simulink model "PreBraking_Scenario1_cs"  (R2014b)
settings: Solver=ode5  SolverMode=SingleTasking  StartTime=0.0  StopTime=inf  FixedStep=1/100  RelTol=1e-3
PreLoadFcn:
  | mbxruntime.callbacks.PreLoadFcn(bdroot);
  | check_NUTS_defined;
  | 
  | assignin('base',['model_closed_' bdroot],false);addpath('../includes_AEBS');
PostLoadFcn:
  | mbxruntime.callbacks.PostLoadFcn(bdroot);
InitFcn:
  | mbxruntime.callbacks.InitFcn(bdroot);
StartFcn:
  | mbxruntime.callbacks.StartFcn(bdroot);
StopFcn:
  | mbxruntime.callbacks.StopFcn(bdroot);
model workspace: external: MAT-File .\PreBraking_Scenario1_cs_hws.mat (data not in the file)
undefined symbols (not defined in the file or in its folder): OrientationPitch, OrientationRoll, PositionX, PositionY, PositionZ, warningInitialVelocity, x0
undefined symbols (not defined in the file): PreBraking_Scenario1_cs_026d0cdcec288b62, PreBraking_Scenario1_cs_0385b51e7df15a58, PreBraking_Scenario1_cs_0b30baef7b6532db, PreBraking_Scenario1_cs_0d6875a57991286b, PreBraking_Scenario1_cs_138be516424db58b, PreBraking_Scenario1_cs_23d3d4fc5b63e353, PreBraking_Scenario1_cs_2f0f014f8afaa95e, PreBraking_Scenario1_cs_37a5b238ce9b9d58, PreBraking_Scenario1_cs_3e434e556dc94cce, PreBraking_Scenario1_cs_46f0ee8501fe1889, PreBraking_Scenario1_cs_5d62597554acff95, PreBraking_Scenario1_cs_5da0fc6e87d9d5b3, PreBraking_Scenario1_cs_5ed65167116c3469, PreBraking_Scenario1_cs_6eb9f15635d94d0c, PreBraking_Scenario1_cs_783b9a4fac440b07, PreBraking_Scenario1_cs_7a7290d742a44883, PreBraking_Scenario1_cs_82e3a60ee2034171, PreBraking_Scenario1_cs_8b2784fe49c992e6, PreBraking_Scenario1_cs_9206a2e3911d44de, PreBraking_Scenario1_cs_983f811fe80a5f0d, PreBraking_Scenario1_cs_9b466beab5d2337e, PreBraking_Scenario1_cs_a08e42c00c044b50, PreBraking_Scenario1_cs_Audi_A8_1_Dynamics_Simple_initialPitch, PreBraking_Scenario1_cs_Audi_A8_1_Dynamics_Simple_initialRoll, PreBraking_Scenario1_cs_Audi_A8_1_Dynamics_Simple_initialX, PreBraking_Scenario1_cs_Audi_A8_1_Dynamics_Simple_initialY, PreBraking_Scenario1_cs_Audi_A8_1_Dynamics_Simple_initialYaw, PreBraking_Scenario1_cs_Audi_A8_1_Dynamics_Simple_initialZ, PreBraking_Scenario1_cs_b7d11204e3bec466, PreBraking_Scenario1_cs_c7aafe2117783533, PreBraking_Scenario1_cs_cbbde59a5a2cb59b, PreBraking_Scenario1_cs_ccf63f357a330662, PreBraking_Scenario1_cs_Citroen_C3_3_Path_pathUniqueID, PreBraking_Scenario1_cs_d4efba4491f01d46, PreBraking_Scenario1_cs_d59dc65fc07c1f25, PreBraking_Scenario1_cs_d8dfcf69a768aef8, PreBraking_Scenario1_cs_dcfa2001fd35d12a, PreBraking_Scenario1_cs_eaed30225f637059, PreBraking_Scenario1_cs_ecfe80b42161c93b, PreBraking_Scenario1_cs_f61ea707e711400d, PreBraking_Scenario1_cs_Toyota_Previa_1_Path_pathUniqueID, SteeringColumn, SteeringWheel, WheelL0, WheelL1, WheelR0, WheelR1
libraries: simulink_extras x41, simulink x20, PreScanSimulinkLibrary x13, PreScanUsefulBlocks x2
(part 1 of 14)
CloseFcn:
  | mbxruntime.callbacks.CloseFcn(bdroot);
  | evalin('base',['clear model_closed_' bdroot]);
settings Model: Creator=PRESCAN  LastModifiedBy=jenkins
settings DataIOCC: SignalLoggingSaveFormat=ModelDataLogs
settings OptimizationCC: InlineParams=on  ExpressionDepthLimit=2147483647  InitFltsAndDblsToZero=on
settings DebuggingCC: SaveWithParameterizedLinksMsg=none  UnderspecifiedInitializationDetection=Classic  MergeDetectMultiDrivingBlocksExec=none  SignalResolutionControl=TryResolveAllWithWarning  SolverPrmCheckMsg=none  MultiTaskDSMMsg=warning  MultiTaskCondExecSysMsg=none  FcnCallInpInsideContextMsg=UseLocalSettings  StateNameClashWarn=warning
settings ModelReferenceCC: UpdateModelReferenceTargets=IfOutOfDate
settings SFSimCC: SimParseCustomCode=off
settings SFSimCC: SimCustomHeaderCode=|
  | #include "prescan_collisiondetection_data.h"
  | #include "prescan.h"
  | #include "prescan_platform.h"
settings RTWCC: IncludeERTFirstTime=on
settings GRTTargetCC: TargetFcnLib=ansi_tfl_tmw.mat  CombineOutputUpdateFcns=off  GRTInterface=on

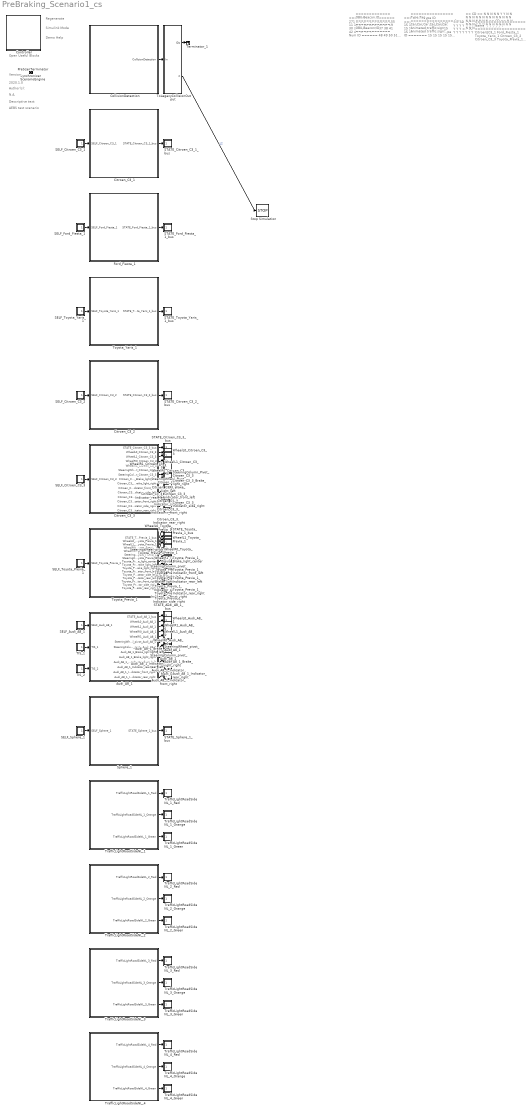
== system PreBraking_Scenario1_cs ==
  note: Regenerate
  note: Simulink Mode
  note: Open Useful Blocks
  note: 2020.1.0
  note: Version:
  note: Author(s):
  note: N.A.
  note: Descriptive text:
  note: AEBS test scenario
  note: Demo Help
  note: ======
      | Num ID
      | ======
      | 271
      | 272
      | 274
      | 276
      | 152
      | 18
      | 155
      | 11
      | 13
      | 14
      | 15
      | 21
      | 24
      | 26
      | 27
      | 29
      | 30
      | 31
      | 32
      | 33
      | 34
      | 35
      | 37
      | 38
      | 41
      | 42
      | 44
      | 45
      | 46
      | 47
      | ======
      | Num ID
      | ======
      | 48
      | 49
      | 50
      | 51
      | 52
      | 54
      | 55
      | 180
      | 188
      | 196
      | 204
      | 210
      | 218
      | 226
      | 234
      | 579
      | 586
      | 591
      | 154
  note: =============
      | OBU-Beacon ID
      | =============
      |
      |
      |
      |
      |
      |
      |
      |
      |
      |
      |
      |
      |
      |
      |
      |
      |
      |
      |
      |
      |
      |
      |
      |
      |
      |
      |
      |
      |
      |
      | =============
      | OBU-Beacon ID
      | =============
  note: =======
      | Type ID
      | =======
      | 1
      | 1
      | 1
      | 1
      | 1
      | 1
      | 1
      | 15
      | 15
      | 15
      | 15
      | 15
      | 15
      | 15
      | 15
      | 15
      | 15
      | 15
      | 15
      | 15
      | 15
      | 15
      | 15
      | 15
      | 15
      | 15
      | 15
      | 15
      | 15
      | 15
      | =======
      | Type ID
      | =======
      | 15
      | 15
      | 15
      | 15
      | 15
      | 15
      | 15
      | 13
      | 13
      | 13
      | 13
      | 13
      | 13
      | 13
      | 13
      | 13
      | 13
      | 13
      | 13
  note: ================
      | Type Tag
      | ================
      | Car
      | Car
      | Car
      | Car
      | Car
      | Car
      | Car
      | Animated traffic sign
      | Animated traffic sign
      | Animated traffic sign
      | Animated traffic sign
      | Animated traffic sign
      | Animated traffic sign
      | Animated traffic sign
      | Animated traffic sign
      | Animated traffic sign
      | Animated traffic sign
      | Animated traffic sign
      | Animated traffic sign
      | Animated traffic sign
      | Animated traffic sign
      | Animated traffic sign
      | Animated traffic sign
      | Animated traffic sign
      | Animated traffic sign
      | Animated traffic sign
      | Animated traffic sign
      | Animated traffic sign
      | Animated traffic sign
      | Animated traffic sign
      | ================
      | Type Tag
      | ================
      | Animated traffic sign
      | Animated traffic sign
      | Animated traffic sign
      | Animated traffic sign
      | Animated traffic sign
      | Animated traffic sign
      | Animated traffic sign
      | Natural element
      | Natural element
      | Natural element
      | Natural element
      | Natural element
      | Natural element
      | Natural element
      | Natural element
      | Natural element
      | Natural element
      | Natural element
      | Natural element
  note: ==
      | SD
      | ==
      | Y
      | Y
      | Y
      | Y
      | Y
      | Y
      | Y
      | Y
      | Y
      | Y
      | Y
      | Y
      | Y
      | Y
      | Y
      | Y
      | Y
      | Y
      | Y
      | Y
      | Y
      | Y
      | Y
      | Y
      | Y
      | Y
      | Y
      | Y
      | Y
      | Y
      | ==
      | SD
      | ==
      | Y
      | Y
      | Y
      | Y
      | Y
      | Y
      | Y
      | Y
      | Y
      | Y
      | Y
      | Y
      | Y
      | Y
      | Y
      | Y
      | Y
      | Y
      | Y
  note: ==
      | CD
      | ==
      | N
      | N
      | N
      | N
      | N
      | Y
      | Y
      | N
      | N
      | N
      | N
      | N
      | N
      | N
      | N
      | N
      | N
      | N
      | N
      | N
      | N
      | N
      | N
      | N
      | N
      | N
      | N
      | N
      | N
      | N
      | ==
      | CD
      | ==
      | N
      | N
      | N
      | N
      | N
      | N
      | N
      | N
      | N
      | N
      | N
      | N
      | N
      | N
      | N
      | N
      | N
      | N
      | N
  note: ===================
      | Name
      | ===================
      | Citroen_C3_1
      | Ford_Fiesta_1
      | Toyota_Yaris_1
      | Citroen_C3_2
      | Citroen_C3_3
      | Toyota_Previa_1
      | Audi_A8_1
      | TrafficLightRoadSideNL_1
      | TrafficLightRoadSideNL_2
      | TrafficLightRoadSideNL_3
      | TrafficLightRoadSideNL_4
      | Lightpost_1
      | Lightpost_3
      | Lightpost_5
      | Lightpost_6
      | Lightpost_8
      | Lightpost_9
      | Lightpost_10
      | Lightpost_11
      | Lightpost_12
      | Lightpost_13
      | Lightpost_14
      | Lightpost_16
      | Lightpost_17
      | Lightpost_20
      | Lightpost_21
      | Lightpost_23
      | Lightpost_24
      | Lightpost_25
      | Lightpost_26
      | ===================
      | Name
      | ===================
      | Lightpost_27
      | Lightpost_28
      | Lightpost_29
      | Lightpost_30
      | Lightpost_31
      | Lightpost_33
      | Lightpost_34
      | ServiceBerry_Age12_31
      | ServiceBerry_Age12_39
      | ServiceBerry_Age12_47
      | ServiceBerry_Age12_55
      | ServiceBerry_Age12_61
      | ServiceBerry_Age12_69
      | ServiceBerry_Age12_77
      | ServiceBerry_Age12_85
      | ServiceBerry_Age12_430
      | ServiceBerry_Age12_437
      | ServiceBerry_Age12_442
      | Magnolia_Age10_1
  Audi_A8_1 : Subsystem  Tag=WorldObjectSubSystem  InitFcn=UniqueId = '1001';
      mask init:
      | modelPath = GenericModelHelper.getGenericModelFilePath('ModelDepo','Vehicles\Audi_A8\Audi_A8.pgmb','e33fe1ddcf3e8ae97caccbc8f2fa74ac');imagePath = GenericModelHelper.getCompilationPicture(modelPath, 'Audi_A8_HighPoly.png');
      mask Display: image(imread(imagePath));color('white');text(0, 0, ' ID=155\n')
  Audi_A8_1_Brake_light_left : Subsystem  Tag=actuator/BrakeLightL  Priority=0  LoadFcn=load('PreScanVisuLightActuatorData');load('PrescanRPYData');load('PrescanXYZData');load('PreScanRGBData')  mask(PreScan Sink Block: VisuActiveLight){}
      mask help:
      | The VisuActiveLight block provides a way for detailed animation of Light Sources, such as the indicator, brake, fog and main lights of a vehicle, or a light post.
      |
      | For more information, please click Help.
      settings: OpenFcn=open_system([gcb '/Actuator'],'mask')
      mask Help: eval('openHelp(209)')
      mask Display: image(imread('HeadLight.png'))
  Audi_A8_1_Brake_light_right : Subsystem  Tag=actuator/BrakeLightR  Priority=0  LoadFcn=load('PreScanVisuLightActuatorData');load('PrescanRPYData');load('PrescanXYZData');load('PreScanRGBData')  mask(PreScan Sink Block: VisuActiveLight){}
      mask help:
      | The VisuActiveLight block provides a way for detailed animation of Light Sources, such as the indicator, brake, fog and main lights of a vehicle, or a light post.
      |
      | For more information, please click Help.
      settings: OpenFcn=open_system([gcb '/Actuator'],'mask')
      mask Help: eval('openHelp(209)')
      mask Display: image(imread('HeadLight.png'))
  Audi_A8_1_Indicator_front_left : Subsystem  Tag=actuator/IndicatorFL  Priority=0  LoadFcn=load('PreScanVisuLightActuatorData');load('PrescanRPYData');load('PrescanXYZData');load('PreScanRGBData')  mask(PreScan Sink Block: VisuActiveLight){}
      mask help:
      | The VisuActiveLight block provides a way for detailed animation of Light Sources, such as the indicator, brake, fog and main lights of a vehicle, or a light post.
      |
      | For more information, please click Help.
      settings: OpenFcn=open_system([gcb '/Actuator'],'mask')
      mask Help: eval('openHelp(209)')
      mask Display: image(imread('HeadLight.png'))
  Audi_A8_1_Indicator_front_right : Subsystem  Tag=actuator/IndicatorFR  Priority=0  LoadFcn=load('PreScanVisuLightActuatorData');load('PrescanRPYData');load('PrescanXYZData');load('PreScanRGBData')  mask(PreScan Sink Block: VisuActiveLight){}
      mask help:
      | The VisuActiveLight block provides a way for detailed animation of Light Sources, such as the indicator, brake, fog and main lights of a vehicle, or a light post.
      |
      | For more information, please click Help.
      settings: OpenFcn=open_system([gcb '/Actuator'],'mask')
      mask Help: eval('openHelp(209)')
      mask Display: image(imread('HeadLight.png'))
  Audi_A8_1_Indicator_rear_left : Subsystem  Tag=actuator/IndicatorRL  Priority=0  LoadFcn=load('PreScanVisuLightActuatorData');load('PrescanRPYData');load('PrescanXYZData');load('PreScanRGBData')  mask(PreScan Sink Block: VisuActiveLight){}
      mask help:
      | The VisuActiveLight block provides a way for detailed animation of Light Sources, such as the indicator, brake, fog and main lights of a vehicle, or a light post.
      |
      | For more information, please click Help.
      settings: OpenFcn=open_system([gcb '/Actuator'],'mask')
      mask Help: eval('openHelp(209)')
      mask Display: image(imread('HeadLight.png'))
  Audi_A8_1_Indicator_rear_right : Subsystem  Tag=actuator/IndicatorRR  Priority=0  LoadFcn=load('PreScanVisuLightActuatorData');load('PrescanRPYData');load('PrescanXYZData');load('PreScanRGBData')  mask(PreScan Sink Block: VisuActiveLight){}
      mask help:
      | The VisuActiveLight block provides a way for detailed animation of Light Sources, such as the indicator, brake, fog and main lights of a vehicle, or a light post.
      |
      | For more information, please click Help.
      settings: OpenFcn=open_system([gcb '/Actuator'],'mask')
      mask Help: eval('openHelp(209)')
      mask Display: image(imread('HeadLight.png'))
  Citroen_C3_1 : Subsystem  Tag=WorldObjectSubSystem  InitFcn=UniqueId = '978';
      mask init:
      | modelPath = GenericModelHelper.getGenericModelFilePath('ModelDepo','Vehicles\Citroen_C3\Citroen_C3.pgmb','e804ced06d50dbfc6a2202ab3ad01b0c');imagePath = GenericModelHelper.getCompilationPicture(modelPath, 'Citroen_C3_HighPoly.png');
      mask Display: image(imread(imagePath));color('white');text(0, 0, ' ID=271\n')
  Citroen_C3_2 : Subsystem  Tag=WorldObjectSubSystem  InitFcn=UniqueId = '981';
      mask init: same as PreBraking_Scenario1_cs/Citroen_C3_1
      mask Display: image(imread(imagePath));color('white');text(0, 0, ' ID=276\n')
  Citroen_C3_3 : Subsystem  Tag=WorldObjectSubSystem  InitFcn=UniqueId = '987';
      mask init: same as PreBraking_Scenario1_cs/Citroen_C3_1
      mask Display: image(imread(imagePath));color('white');text(0, 0, ' ID=152\n')
  Citroen_C3_3_Brake_light_left : Subsystem  Tag=actuator/BrakeLightL_Pivot  Priority=0  LoadFcn=load('PreScanVisuLightActuatorData');load('PrescanRPYData');load('PrescanXYZData');load('PreScanRGBData')  mask(PreScan Sink Block: VisuActiveLight){}
      mask help:
      | The VisuActiveLight block provides a way for detailed animation of Light Sources, such as the indicator, brake, fog and main lights of a vehicle, or a light post.
      |
      | For more information, please click Help.
      settings: OpenFcn=open_system([gcb '/Actuator'],'mask')
      mask Help: eval('openHelp(209)')
      mask Display: image(imread('HeadLight.png'))
  Citroen_C3_3_Brake_light_right : Subsystem  Tag=actuator/BrakeLightR_Pivot  Priority=0  LoadFcn=load('PreScanVisuLightActuatorData');load('PrescanRPYData');load('PrescanXYZData');load('PreScanRGBData')  mask(PreScan Sink Block: VisuActiveLight){}
      mask help:
      | The VisuActiveLight block provides a way for detailed animation of Light Sources, such as the indicator, brake, fog and main lights of a vehicle, or a light post.
      |
      | For more information, please click Help.
      settings: OpenFcn=open_system([gcb '/Actuator'],'mask')
      mask Help: eval('openHelp(209)')
      mask Display: image(imread('HeadLight.png'))
  Citroen_C3_3_Indicator_front_left : Subsystem  Tag=actuator/IndicatorFL_Pivot  Priority=0  LoadFcn=load('PreScanVisuLightActuatorData');load('PrescanRPYData');load('PrescanXYZData');load('PreScanRGBData')  mask(PreScan Sink Block: VisuActiveLight){}
      mask help:
      | The VisuActiveLight block provides a way for detailed animation of Light Sources, such as the indicator, brake, fog and main lights of a vehicle, or a light post.
      |
      | For more information, please click Help.
      settings: OpenFcn=open_system([gcb '/Actuator'],'mask')
      mask Help: eval('openHelp(209)')
      mask Display: image(imread('HeadLight.png'))
  Citroen_C3_3_Indicator_front_right : Subsystem  Tag=actuator/IndicatorFR_Pivot  Priority=0  LoadFcn=load('PreScanVisuLightActuatorData');load('PrescanRPYData');load('PrescanXYZData');load('PreScanRGBData')  mask(PreScan Sink Block: VisuActiveLight){}
      mask help:
      | The VisuActiveLight block provides a way for detailed animation of Light Sources, such as the indicator, brake, fog and main lights of a vehicle, or a light post.
      |
      | For more information, please click Help.
      settings: OpenFcn=open_system([gcb '/Actuator'],'mask')
      mask Help: eval('openHelp(209)')
      mask Display: image(imread('HeadLight.png'))
  Citroen_C3_3_Indicator_rear_left : Subsystem  Tag=actuator/IndicatorRL_Pivot  Priority=0  LoadFcn=load('PreScanVisuLightActuatorData');load('PrescanRPYData');load('PrescanXYZData');load('PreScanRGBData')  mask(PreScan Sink Block: VisuActiveLight){}
      mask help:
      | The VisuActiveLight block provides a way for detailed animation of Light Sources, such as the indicator, brake, fog and main lights of a vehicle, or a light post.
      |
      | For more information, please click Help.
      settings: OpenFcn=open_system([gcb '/Actuator'],'mask')
      mask Help: eval('openHelp(209)')
      mask Display: image(imread('HeadLight.png'))
  Citroen_C3_3_Indicator_rear_right : Subsystem  Tag=actuator/IndicatorRR_Pivot  Priority=0  LoadFcn=load('PreScanVisuLightActuatorData');load('PrescanRPYData');load('PrescanXYZData');load('PreScanRGBData')  mask(PreScan Sink Block: VisuActiveLight){}
      mask help:
      | The VisuActiveLight block provides a way for detailed animation of Light Sources, such as the indicator, brake, fog and main lights of a vehicle, or a light post.
      |
      | For more information, please click Help.
      settings: OpenFcn=open_system([gcb '/Actuator'],'mask')
      mask Help: eval('openHelp(209)')
      mask Display: image(imread('HeadLight.png'))
  Citroen_C3_3_Indicator_side_left : Subsystem  Tag=actuator/IndicatorSL_Pivot  Priority=0  LoadFcn=load('PreScanVisuLightActuatorData');load('PrescanRPYData');load('PrescanXYZData');load('PreScanRGBData')  mask(PreScan Sink Block: VisuActiveLight){}
      mask help:
      | The VisuActiveLight block provides a way for detailed animation of Light Sources, such as the indicator, brake, fog and main lights of a vehicle, or a light post.
      |
      | For more information, please click Help.
      settings: OpenFcn=open_system([gcb '/Actuator'],'mask')
      mask Help: eval('openHelp(209)')
      mask Display: image(imread('HeadLight.png'))
  Citroen_C3_3_Indicator_side_right : Subsystem  Tag=actuator/IndicatorSR_Pivot  Priority=0  LoadFcn=load('PreScanVisuLightActuatorData');load('PrescanRPYData');load('PrescanXYZData');load('PreScanRGBData')  mask(PreScan Sink Block: VisuActiveLight){}
      mask help:
      | The VisuActiveLight block provides a way for detailed animation of Light Sources, such as the indicator, brake, fog and main lights of a vehicle, or a light post.
      |
      | For more information, please click Help.
      settings: OpenFcn=open_system([gcb '/Actuator'],'mask')
      mask Help: eval('openHelp(209)')
      mask Display: image(imread('HeadLight.png'))
  CollisionDetection : Subsystem  Tag=sensor/CollisionDetection  Priority=30  LoadFcn=load('PrescanCollisionDetectionData.mat');load('PrescanCollisionDetectionMessage.mat')  mask(PreScan Source Block: CollisionDetection){}
      mask help: Collision Detection can be used to detect collisions between PreScan components. For Collision Detection the actual component shape is taken into account, so it is not a bounding box approach.
      settings: OpenFcn=open_system([gcb '/Sensor'],'mask')
      mask Help: eval('openHelp(811)')
      mask Display: image(imread('crash.jpg'))
  Controller : Subsystem  Description=8A3CD2955739A82C886C20AE3E253D78460D53180EE2C1B14CC08DF75A70BE77  Priority=-1  LoadFcn=load PreScanControllerData  mask(PreScan Simulation Controller){prescanversion='2020.1.0', ModelReferencing=off, TimeStep=1/100, ControlMode=0, PreScanExecutionMode=on, ControllerCount=0, ControllerIndex=0, ControllerOptions=''}
      mask prompts: prescanversion "PreScan Version"; ModelReferencing "Use Model Referencing"; TimeStep "Upload Period [s]"; ControlMode "Control Mode"; PreScanExecutionMode "Execution Mode"; ControllerCount "Controller Count"; ControllerIndex "Controller Index"; ControllerOptions "Controller Options"
      mask help:
      | Please do not remove this block from the compilation sheet,
      | as it connects the model to the PreScan environment.
      mask init:
      | model = bdroot(gcb);
      | ExperimentFile = mbxruntime.findExperimentFile(model,true); %relative path
      | 
      | [d1, d2, d3, prescandata] = prescan_Settings();
      | ModelDepo = fullfile(prescandata,'ModelDepo'); 
      | 
      | RTmode = mbxruntime.getRTMode(model);
      | 
      | SimulationMode = get_param(bdroot,'SimulationMode');
      | if strcmp(SimulationMode, 'rapid-accelerator')
      |     SimulationMode = 'external';
      | end
      | TargetName = get_param(bdroot,'SystemTargetFile');
      settings: ModelCloseFcn=assignin('base',['model_closed_' bdroot],true);
      mask Help: eval('openHelp(812)')
      mask Display: image(imread('prescanlogo.ico'))
  Ford_Fiesta_1 : Subsystem  Tag=WorldObjectSubSystem  InitFcn=UniqueId = '979';
      mask init:
      | modelPath = GenericModelHelper.getGenericModelFilePath('ModelDepo','Vehicles\Ford_Fiesta\Ford_Fiesta.pgmb','fe2c7a73e0a60cba76689b71cd1bb76a');imagePath = GenericModelHelper.getCompilationPicture(modelPath, 'Ford_Fiesta_HighPoly.png');
      mask Display: image(imread(imagePath));color('white');text(0, 0, ' ID=272\n')
  PreScanTerminator : Subsystem  Tag=PreScanTerminator  Priority=999  LoadFcn=load PrescanTerminatorData  mask(PreScan Simulation Terminator){TimeStep=1/100}
      mask prompts: TimeStep "Upload Period [s]"
      mask help:
      | Please do not remove this block from the compilation sheet as it
      | connects the model to the PreScan environment.
      mask Help: eval('openHelp(812)')
      mask Display: image(imread('prescanlogo.ico'))
  SELF_Audi_A8_1 : Subsystem  Tag=sensor/SelfPort  Priority=30  LoadFcn=load('PreScanSelfSensorData.mat')  mask(PreScan Source Block: SELF){}
      mask help:
      | The SELF port shows (state) information of the actor itself. The outputs are position in the experiment's axis system and the GPS coordinates, and the object's absolute velocity and compass heading.
      |
      | For more information, please click Help.
      settings: OpenFcn=open_system([gcb '/Sensor'],'mask')
      mask Help: eval('openHelp(462)')
      mask Display: image(imread('GPS.png'))
  SELF_Citroen_C3_1 : Subsystem  Tag=sensor/SelfPort  Priority=30  LoadFcn=load('PreScanSelfSensorData.mat')  mask(PreScan Source Block: SELF){}
      mask help:
      | The SELF port shows (state) information of the actor itself. The outputs are position in the experiment's axis system and the GPS coordinates, and the object's absolute velocity and compass heading.
      |
      | For more information, please click Help.
      settings: OpenFcn=open_system([gcb '/Sensor'],'mask')
      mask Help: eval('openHelp(462)')
      mask Display: image(imread('GPS.png'))
  SELF_Citroen_C3_2 : Subsystem  Tag=sensor/SelfPort  Priority=30  LoadFcn=load('PreScanSelfSensorData.mat')  mask(PreScan Source Block: SELF){}
      mask help:
      | The SELF port shows (state) information of the actor itself. The outputs are position in the experiment's axis system and the GPS coordinates, and the object's absolute velocity and compass heading.
      |
      | For more information, please click Help.
      settings: OpenFcn=open_system([gcb '/Sensor'],'mask')
      mask Help: eval('openHelp(462)')
      mask Display: image(imread('GPS.png'))
  SELF_Citroen_C3_3 : Subsystem  Tag=sensor/SelfPort  Priority=30  LoadFcn=load('PreScanSelfSensorData.mat')  mask(PreScan Source Block: SELF){}
      mask help:
      | The SELF port shows (state) information of the actor itself. The outputs are position in the experiment's axis system and the GPS coordinates, and the object's absolute velocity and compass heading.
      |
      | For more information, please click Help.
      settings: OpenFcn=open_system([gcb '/Sensor'],'mask')
      mask Help: eval('openHelp(462)')
      mask Display: image(imread('GPS.png'))
  SELF_Ford_Fiesta_1 : Subsystem  Tag=sensor/SelfPort  Priority=30  LoadFcn=load('PreScanSelfSensorData.mat')  mask(PreScan Source Block: SELF){}
      mask help:
      | The SELF port shows (state) information of the actor itself. The outputs are position in the experiment's axis system and the GPS coordinates, and the object's absolute velocity and compass heading.
      |
      | For more information, please click Help.
      settings: OpenFcn=open_system([gcb '/Sensor'],'mask')
      mask Help: eval('openHelp(462)')
      mask Display: image(imread('GPS.png'))
  SELF_Sphere_1 : Subsystem  Tag=sensor/SelfPort  Priority=30  LoadFcn=load('PreScanSelfSensorData.mat')  mask(PreScan Source Block: SELF){}
      mask help:
      | The SELF port shows (state) information of the actor itself. The outputs are position in the experiment's axis system and the GPS coordinates, and the object's absolute velocity and compass heading.
      |
      | For more information, please click Help.
      settings: OpenFcn=open_system([gcb '/Sensor'],'mask')
      mask Help: eval('openHelp(462)')
      mask Display: image(imread('GPS.png'))
  SELF_Toyota_Previa_1 : Subsystem  Tag=sensor/SelfPort  Priority=30  LoadFcn=load('PreScanSelfSensorData.mat')  mask(PreScan Source Block: SELF){}
      mask help:
      | The SELF port shows (state) information of the actor itself. The outputs are position in the experiment's axis system and the GPS coordinates, and the object's absolute velocity and compass heading.
      |
      | For more information, please click Help.
      settings: OpenFcn=open_system([gcb '/Sensor'],'mask')
      mask Help: eval('openHelp(462)')
      mask Display: image(imread('GPS.png'))
  SELF_Toyota_Yaris_1 : Subsystem  Tag=sensor/SelfPort  Priority=30  LoadFcn=load('PreScanSelfSensorData.mat')  mask(PreScan Source Block: SELF){}
      mask help:
      | The SELF port shows (state) information of the actor itself. The outputs are position in the experiment's axis system and the GPS coordinates, and the object's absolute velocity and compass heading.
      |
      | For more information, please click Help.
      settings: OpenFcn=open_system([gcb '/Sensor'],'mask')
      mask Help: eval('openHelp(462)')
      mask Display: image(imread('GPS.png'))
  STATE_Audi_A8_1_bus : Subsystem  Tag=actuator/StatePort  Priority=0  LoadFcn=load('PreScanStateActuatorData.mat')  mask(PreScan Sink Block: State){}
      mask help:
      | The Actor State contains a vector signal of size (9x1), containing the following signals:
      |
      | -  Position    	(x,y,z)             	[m]
      | -  Velocity    	(vx,vy,vz)         	[m/s]
      | -  Angles       	(Roll, Pitch, Yaw)	[rad]
      |
      | The Actor state is defined in the global axis system.
      | The state is superponed on the Initial position defined in the GUI.
      |
      | For more information, please click Help.
      settings: OpenFcn=open_system([gcb '/Actuator'],'mask')
      mask Help: eval('openHelp(222)')
      mask Display: image(imread('State.png'))
  STATE_Citroen_C3_1_bus : Subsystem  Tag=actuator/StatePort  Priority=0  LoadFcn=load('PreScanStateActuatorData.mat')  mask(PreScan Sink Block: State){}
      mask help:
      | The Actor State contains a vector signal of size (9x1), containing the following signals:
      |
      | -  Position    	(x,y,z)             	[m]
      | -  Velocity    	(vx,vy,vz)         	[m/s]
      | -  Angles       	(Roll, Pitch, Yaw)	[rad]
      |
      | The Actor state is defined in the global axis system.
      | The state is superponed on the Initial position defined in the GUI.
      |
      | For more information, please click Help.
      settings: OpenFcn=open_system([gcb '/Actuator'],'mask')
      mask Help: eval('openHelp(222)')
      mask Display: image(imread('State.png'))
  STATE_Citroen_C3_2_bus : Subsystem  Tag=actuator/StatePort  Priority=0  LoadFcn=load('PreScanStateActuatorData.mat')  mask(PreScan Sink Block: State){}
      mask help:
      | The Actor State contains a vector signal of size (9x1), containing the following signals:
      |
      | -  Position    	(x,y,z)             	[m]
      | -  Velocity    	(vx,vy,vz)         	[m/s]
      | -  Angles       	(Roll, Pitch, Yaw)	[rad]
      |
      | The Actor state is defined in the global axis system.
      | The state is superponed on the Initial position defined in the GUI.
      |
      | For more information, please click Help.
      settings: OpenFcn=open_system([gcb '/Actuator'],'mask')
      mask Help: eval('openHelp(222)')
      mask Display: image(imread('State.png'))
  STATE_Citroen_C3_3_bus : Subsystem  Tag=actuator/StatePort  Priority=0  LoadFcn=load('PreScanStateActuatorData.mat')  mask(PreScan Sink Block: State){}
      mask help:
      | The Actor State contains a vector signal of size (9x1), containing the following signals:
      |
      | -  Position    	(x,y,z)             	[m]
      | -  Velocity    	(vx,vy,vz)         	[m/s]
      | -  Angles       	(Roll, Pitch, Yaw)	[rad]
      |
      | The Actor state is defined in the global axis system.
      | The state is superponed on the Initial position defined in the GUI.
      |
      | For more information, please click Help.
      settings: OpenFcn=open_system([gcb '/Actuator'],'mask')
      mask Help: eval('openHelp(222)')
      mask Display: image(imread('State.png'))
  STATE_Ford_Fiesta_1_bus : Subsystem  Tag=actuator/StatePort  Priority=0  LoadFcn=load('PreScanStateActuatorData.mat')  mask(PreScan Sink Block: State){}
      mask help:
      | The Actor State contains a vector signal of size (9x1), containing the following signals:
      |
      | -  Position    	(x,y,z)             	[m]
      | -  Velocity    	(vx,vy,vz)         	[m/s]
      | -  Angles       	(Roll, Pitch, Yaw)	[rad]
      |
      | The Actor state is defined in the global axis system.
      | The state is superponed on the Initial position defined in the GUI.
      |
      | For more information, please click Help.
      settings: OpenFcn=open_system([gcb '/Actuator'],'mask')
      mask Help: eval('openHelp(222)')
      mask Display: image(imread('State.png'))
  STATE_Sphere_1_bus : Subsystem  Tag=actuator/StatePort  Priority=0  LoadFcn=load('PreScanStateActuatorData.mat')  mask(PreScan Sink Block: State){}
      mask help:
      | The Actor State contains a vector signal of size (9x1), containing the following signals:
      |
      | -  Position    	(x,y,z)             	[m]
      | -  Velocity    	(vx,vy,vz)         	[m/s]
      | -  Angles       	(Roll, Pitch, Yaw)	[rad]
      |
      | The Actor state is defined in the global axis system.
      | The state is superponed on the Initial position defined in the GUI.
      |
      | For more information, please click Help.
      settings: OpenFcn=open_system([gcb '/Actuator'],'mask')
      mask Help: eval('openHelp(222)')
      mask Display: image(imread('State.png'))
  STATE_Toyota_Previa_1_bus : Subsystem  Tag=actuator/StatePort  Priority=0  LoadFcn=load('PreScanStateActuatorData.mat')  mask(PreScan Sink Block: State){}
      mask help:
      | The Actor State contains a vector signal of size (9x1), containing the following signals:
      |
      | -  Position    	(x,y,z)             	[m]
      | -  Velocity    	(vx,vy,vz)         	[m/s]
      | -  Angles       	(Roll, Pitch, Yaw)	[rad]
      |
      | The Actor state is defined in the global axis system.
      | The state is superponed on the Initial position defined in the GUI.
      |
      | For more information, please click Help.
      settings: OpenFcn=open_system([gcb '/Actuator'],'mask')
      mask Help: eval('openHelp(222)')
      mask Display: image(imread('State.png'))
  STATE_Toyota_Yaris_1_bus : Subsystem  Tag=actuator/StatePort  Priority=0  LoadFcn=load('PreScanStateActuatorData.mat')  mask(PreScan Sink Block: State){}
      mask help:
      | The Actor State contains a vector signal of size (9x1), containing the following signals:
      |
      | -  Position    	(x,y,z)             	[m]
      | -  Velocity    	(vx,vy,vz)         	[m/s]
      | -  Angles       	(Roll, Pitch, Yaw)	[rad]
      |
      | The Actor state is defined in the global axis system.
      | The state is superponed on the Initial position defined in the GUI.
      |
      | For more information, please click Help.
      settings: OpenFcn=open_system([gcb '/Actuator'],'mask')
      mask Help: eval('openHelp(222)')
      mask Display: image(imread('State.png'))
  ScenarioEngine : Subsystem  Tag=PreScanOpenScenarioBlock  Priority=10  LoadFcn=load PrescanSynchronizeData  mask(PreScan Simulation Core Block){TimeStep=1/100}
      mask prompts: TimeStep "Timestep [s]"
      mask help:
      | Please do not remove this block from the PreScan compilation sheet,
      | as it contains essential configuration parameters for a PreScan simulation.
      settings: DeleteFcn=PreScanBlockDeleteFcn;
      mask Display: image(imread('prescanlogo.ico'))
  Sphere_1 : Subsystem  Tag=WorldObjectSubSystem  InitFcn=UniqueId = '1009';
      mask init:
      | imagePath=which('Sphere.jpg');
      mask Display: image(imread(imagePath));color('white');text(0, 0, ' ID=20\n')
  SteeringColumn_Pivot_Citroen_C3_3 : Subsystem  Tag=Actuator  Priority=0  LoadFcn=load('PrescanPoseData');load('PrescanXYZData');load('PreScanRPYData')
      mask help:
      | The VisuJoint block provides a way to adapt the location and orientation of a part of an object.
      |
      | For more information, please click Help.
      settings: OpenFcn=open_system([gcb '/Actuator'],'mask')
      mask Display: image(imread('Joint.png'))
  SteeringColumn_pivot_Audi_A8_1 : Subsystem  Tag=Actuator  Priority=0  LoadFcn=load('PrescanPoseData');load('PrescanXYZData');load('PreScanRPYData')
      mask help:
      | The VisuJoint block provides a way to adapt the location and orientation of a part of an object.
      |
      | For more information, please click Help.
      settings: OpenFcn=open_system([gcb '/Actuator'],'mask')
      mask Display: image(imread('Joint.png'))
  SteeringColumn_pivot_Toyota_Previa_1 : Subsystem  Tag=Actuator  Priority=0  LoadFcn=load('PrescanPoseData');load('PrescanXYZData');load('PreScanRPYData')
      mask help:
      | The VisuJoint block provides a way to adapt the location and orientation of a part of an object.
      |
      | For more information, please click Help.
      settings: OpenFcn=open_system([gcb '/Actuator'],'mask')
      mask Display: image(imread('Joint.png'))
  SteeringWheel_Pivot_Citroen_C3_3 : Subsystem  Tag=Actuator  Priority=0  LoadFcn=load('PrescanPoseData');load('PrescanXYZData');load('PreScanRPYData')
      mask help:
      | The VisuJoint block provides a way to adapt the location and orientation of a part of an object.
      |
      | For more information, please click Help.
      settings: OpenFcn=open_system([gcb '/Actuator'],'mask')
      mask Display: image(imread('Joint.png'))
  SteeringWheel_pivot_Audi_A8_1 : Subsystem  Tag=Actuator  Priority=0  LoadFcn=load('PrescanPoseData');load('PrescanXYZData');load('PreScanRPYData')
      mask help:
      | The VisuJoint block provides a way to adapt the location and orientation of a part of an object.
      |
      | For more information, please click Help.
      settings: OpenFcn=open_system([gcb '/Actuator'],'mask')
      mask Display: image(imread('Joint.png'))
  SteeringWheel_pivot_Toyota_Previa_1 : Subsystem  Tag=Actuator  Priority=0  LoadFcn=load('PrescanPoseData');load('PrescanXYZData');load('PreScanRPYData')
      mask help:
      | The VisuJoint block provides a way to adapt the location and orientation of a part of an object.
      |
      | For more information, please click Help.
      settings: OpenFcn=open_system([gcb '/Actuator'],'mask')
      mask Display: image(imread('Joint.png'))
  Stop Simulation : Stop
  Synchronizer : Subsystem  Tag=PreScanSynchronizer  Priority=20  LoadFcn=load PrescanSynchronizeData  mask(PreScan Simulation Core Block){TimeStep=1/100}
      mask prompts: TimeStep "Timestep [s]"
      mask help:
      | Please do not remove this block from the PreScan compilation sheet,
      | as it contains essential configuration parameters for a PreScan simulation.
      settings: DeleteFcn=PreScanBlockDeleteFcn;
      mask Display: image(imread('prescanlogo.ico'))
  TIS_1 : Subsystem  Tag=sensor/TIS  Priority=30  LoadFcn=load('PrescanScannerSensorData.mat');load('PrescanScannerSensorMessage.mat')  mask(PreScan Source Block: Technology Independent Sensor (TIS)){}
      mask help:
      | The Technology Independent Sensor (TIS) provides a sensor with all sensor-related influence factors (like noise, drift and accuracy) without being technology specific (like radar and lidar). The TIS detects the closest point on the geometry of an object.
      |
      | For more information, please click Help.
      settings: OpenFcn=open_system([gcb '/Sensor'],'mask')
      mask Help: eval('openHelp(449)')
      mask Display: image(imread('TIS.png'))
  TIS_2 : Subsystem  Tag=sensor/TIS  Priority=30  LoadFcn=load('PrescanScannerSensorData.mat');load('PrescanScannerSensorMessage.mat')  mask(PreScan Source Block: Technology Independent Sensor (TIS)){}
      mask help:
      | The Technology Independent Sensor (TIS) provides a sensor with all sensor-related influence factors (like noise, drift and accuracy) without being technology specific (like radar and lidar). The TIS detects the closest point on the geometry of an object.
      |
      | For more information, please click Help.
      settings: OpenFcn=open_system([gcb '/Sensor'],'mask')
      mask Help: eval('openHelp(449)')
      mask Display: image(imread('TIS.png'))
  Terminator_1 : Terminator
  ToLegacyCollisionOutput : Subsystem  Tag=ToLegacyCollisionOutput
      settings: CopyFcn=load('PrescanCollisionDetectionMessage'); prescanAddSimHeader(bdroot,PRESCAN_COLLISIONDETECTION_MESSAGE);
  Toyota_Previa_1 : Subsystem  Tag=WorldObjectSubSystem  InitFcn=UniqueId = '991';
      mask init:
      | modelPath = GenericModelHelper.getGenericModelFilePath('ModelDepo','Vehicles\Toyota_Previa\Toyota_Previa.pgmb','93e58f95175b34f6ce91a88cdfe55b40');imagePath = GenericModelHelper.getCompilationPicture(modelPath, 'Toyota_Previa_HighPoly.png');
      mask Display: image(imread(imagePath));color('white');text(0, 0, ' ID=18\n')
  Toyota_Previa_1_Brake_light_center : Subsystem  Tag=actuator/BrakeLightM  Priority=0  LoadFcn=load('PreScanVisuLightActuatorData');load('PrescanRPYData');load('PrescanXYZData');load('PreScanRGBData')  mask(PreScan Sink Block: VisuActiveLight){}
      mask help:
      | The VisuActiveLight block provides a way for detailed animation of Light Sources, such as the indicator, brake, fog and main lights of a vehicle, or a light post.
      |
      | For more information, please click Help.
      settings: OpenFcn=open_system([gcb '/Actuator'],'mask')
      mask Help: eval('openHelp(209)')
      mask Display: image(imread('HeadLight.png'))
  Toyota_Previa_1_Brake_light_left : Subsystem  Tag=actuator/BrakeLightL  Priority=0  LoadFcn=load('PreScanVisuLightActuatorData');load('PrescanRPYData');load('PrescanXYZData');load('PreScanRGBData')  mask(PreScan Sink Block: VisuActiveLight){}
      mask help:
      | The VisuActiveLight block provides a way for detailed animation of Light Sources, such as the indicator, brake, fog and main lights of a vehicle, or a light post.
      |
      | For more information, please click Help.
      settings: OpenFcn=open_system([gcb '/Actuator'],'mask')
      mask Help: eval('openHelp(209)')
      mask Display: image(imread('HeadLight.png'))
  Toyota_Previa_1_Brake_light_right : Subsystem  Tag=actuator/BrakeLightR  Priority=0  LoadFcn=load('PreScanVisuLightActuatorData');load('PrescanRPYData');load('PrescanXYZData');load('PreScanRGBData')  mask(PreScan Sink Block: VisuActiveLight){}
      mask help:
      | The VisuActiveLight block provides a way for detailed animation of Light Sources, such as the indicator, brake, fog and main lights of a vehicle, or a light post.
      |
      | For more information, please click Help.
      settings: OpenFcn=open_system([gcb '/Actuator'],'mask')
      mask Help: eval('openHelp(209)')
      mask Display: image(imread('HeadLight.png'))
  Toyota_Previa_1_Indicator_front_left : Subsystem  Tag=actuator/IndicatorFL  Priority=0  LoadFcn=load('PreScanVisuLightActuatorData');load('PrescanRPYData');load('PrescanXYZData');load('PreScanRGBData')  mask(PreScan Sink Block: VisuActiveLight){}
      mask help:
      | The VisuActiveLight block provides a way for detailed animation of Light Sources, such as the indicator, brake, fog and main lights of a vehicle, or a light post.
      |
      | For more information, please click Help.
      settings: OpenFcn=open_system([gcb '/Actuator'],'mask')
      mask Help: eval('openHelp(209)')
      mask Display: image(imread('HeadLight.png'))
  Toyota_Previa_1_Indicator_front_right : Subsystem  Tag=actuator/IndicatorFR  Priority=0  LoadFcn=load('PreScanVisuLightActuatorData');load('PrescanRPYData');load('PrescanXYZData');load('PreScanRGBData')  mask(PreScan Sink Block: VisuActiveLight){}
      mask help:
      | The VisuActiveLight block provides a way for detailed animation of Light Sources, such as the indicator, brake, fog and main lights of a vehicle, or a light post.
      |
      | For more information, please click Help.
      settings: OpenFcn=open_system([gcb '/Actuator'],'mask')
      mask Help: eval('openHelp(209)')
      mask Display: image(imread('HeadLight.png'))
  Toyota_Previa_1_Indicator_rear_left : Subsystem  Tag=actuator/IndicatorRL  Priority=0  LoadFcn=load('PreScanVisuLightActuatorData');load('PrescanRPYData');load('PrescanXYZData');load('PreScanRGBData')  mask(PreScan Sink Block: VisuActiveLight){}
      mask help:
      | The VisuActiveLight block provides a way for detailed animation of Light Sources, such as the indicator, brake, fog and main lights of a vehicle, or a light post.
      |
      | For more information, please click Help.
      settings: OpenFcn=open_system([gcb '/Actuator'],'mask')
      mask Help: eval('openHelp(209)')
      mask Display: image(imread('HeadLight.png'))
  Toyota_Previa_1_Indicator_rear_right : Subsystem  Tag=actuator/IndicatorRR  Priority=0  LoadFcn=load('PreScanVisuLightActuatorData');load('PrescanRPYData');load('PrescanXYZData');load('PreScanRGBData')  mask(PreScan Sink Block: VisuActiveLight){}
      mask help:
      | The VisuActiveLight block provides a way for detailed animation of Light Sources, such as the indicator, brake, fog and main lights of a vehicle, or a light post.
      |
      | For more information, please click Help.
      settings: OpenFcn=open_system([gcb '/Actuator'],'mask')
      mask Help: eval('openHelp(209)')
      mask Display: image(imread('HeadLight.png'))
  Toyota_Previa_1_Indicator_side_left : Subsystem  Tag=actuator/IndicatorSL  Priority=0  LoadFcn=load('PreScanVisuLightActuatorData');load('PrescanRPYData');load('PrescanXYZData');load('PreScanRGBData')  mask(PreScan Sink Block: VisuActiveLight){}
      mask help:
      | The VisuActiveLight block provides a way for detailed animation of Light Sources, such as the indicator, brake, fog and main lights of a vehicle, or a light post.
      |
      | For more information, please click Help.
      settings: OpenFcn=open_system([gcb '/Actuator'],'mask')
      mask Help: eval('openHelp(209)')
      mask Display: image(imread('HeadLight.png'))
  Toyota_Previa_1_Indicator_side_right : Subsystem  Tag=actuator/IndicatorSR  Priority=0  LoadFcn=load('PreScanVisuLightActuatorData');load('PrescanRPYData');load('PrescanXYZData');load('PreScanRGBData')  mask(PreScan Sink Block: VisuActiveLight){}
      mask help:
      | The VisuActiveLight block provides a way for detailed animation of Light Sources, such as the indicator, brake, fog and main lights of a vehicle, or a light post.
      |
      | For more information, please click Help.
      settings: OpenFcn=open_system([gcb '/Actuator'],'mask')
      mask Help: eval('openHelp(209)')
      mask Display: image(imread('HeadLight.png'))
  Toyota_Yaris_1 : Subsystem  Tag=WorldObjectSubSystem  InitFcn=UniqueId = '980';
      mask init:
      | modelPath = GenericModelHelper.getGenericModelFilePath('ModelDepo','Vehicles\Toyota_Yaris\Toyota_Yaris.pgmb','3ea2b9be97d70b5ca322b210574befd9');imagePath = GenericModelHelper.getCompilationPicture(modelPath, 'Toyota_Yaris_HighPoly.png');
      mask Display: image(imread(imagePath));color('white');text(0, 0, ' ID=274\n')
  TrafficLightRoadSideNL_1 : Subsystem  Tag=WorldObjectSubSystem  InitFcn=UniqueId = '26';
      mask init:
      | modelPath = GenericModelHelper.getGenericModelFilePath('ModelDepo','AnimatedElements\TrafficLight_NL\Roadside\Roadside_NL.pgmb','2000fba5e1a6d0fba32e88146243c3cb');imagePath = GenericModelHelper.getCompilationPicture(modelPath, 'Roadside_NL.png');
      mask Display: image(imread(imagePath));color('white');text(0, 0, ' ID=11\n')
  TrafficLightRoadSideNL_1_Green : Subsystem  Tag=actuator/Green  Priority=0  LoadFcn=load('PreScanVisuLightActuatorData');load('PrescanRPYData');load('PrescanXYZData');load('PreScanRGBData')  mask(PreScan Sink Block: VisuActiveLight){}
      mask help:
      | The VisuActiveLight block provides a way for detailed animation of Light Sources, such as the indicator, brake, fog and main lights of a vehicle, or a light post.
      |
      | For more information, please click Help.
      settings: OpenFcn=open_system([gcb '/Actuator'],'mask')
      mask Help: eval('openHelp(209)')
      mask Display: image(imread('HeadLight.png'))
  TrafficLightRoadSideNL_1_Orange : Subsystem  Tag=actuator/Orange  Priority=0  LoadFcn=load('PreScanVisuLightActuatorData');load('PrescanRPYData');load('PrescanXYZData');load('PreScanRGBData')  mask(PreScan Sink Block: VisuActiveLight){}
      mask help:
      | The VisuActiveLight block provides a way for detailed animation of Light Sources, such as the indicator, brake, fog and main lights of a vehicle, or a light post.
      |
      | For more information, please click Help.
      settings: OpenFcn=open_system([gcb '/Actuator'],'mask')
      mask Help: eval('openHelp(209)')
      mask Display: image(imread('HeadLight.png'))
  TrafficLightRoadSideNL_1_Red : Subsystem  Tag=actuator/Red  Priority=0  LoadFcn=load('PreScanVisuLightActuatorData');load('PrescanRPYData');load('PrescanXYZData');load('PreScanRGBData')  mask(PreScan Sink Block: VisuActiveLight){}
      mask help:
      | The VisuActiveLight block provides a way for detailed animation of Light Sources, such as the indicator, brake, fog and main lights of a vehicle, or a light post.
      |
      | For more information, please click Help.
      settings: OpenFcn=open_system([gcb '/Actuator'],'mask')
      mask Help: eval('openHelp(209)')
      mask Display: image(imread('HeadLight.png'))
  TrafficLightRoadSideNL_2 : Subsystem  Tag=WorldObjectSubSystem  InitFcn=UniqueId = '27';
      mask init: same as PreBraking_Scenario1_cs/TrafficLightRoadSideNL_1
      mask Display: image(imread(imagePath));color('white');text(0, 0, ' ID=13\n')
  TrafficLightRoadSideNL_2_Green : Subsystem  Tag=actuator/Green  Priority=0  LoadFcn=load('PreScanVisuLightActuatorData');load('PrescanRPYData');load('PrescanXYZData');load('PreScanRGBData')  mask(PreScan Sink Block: VisuActiveLight){}
      mask help:
      | The VisuActiveLight block provides a way for detailed animation of Light Sources, such as the indicator, brake, fog and main lights of a vehicle, or a light post.
      |
      | For more information, please click Help.
      settings: OpenFcn=open_system([gcb '/Actuator'],'mask')
      mask Help: eval('openHelp(209)')
      mask Display: image(imread('HeadLight.png'))
  TrafficLightRoadSideNL_2_Orange : Subsystem  Tag=actuator/Orange  Priority=0  LoadFcn=load('PreScanVisuLightActuatorData');load('PrescanRPYData');load('PrescanXYZData');load('PreScanRGBData')  mask(PreScan Sink Block: VisuActiveLight){}
      mask help:
      | The VisuActiveLight block provides a way for detailed animation of Light Sources, such as the indicator, brake, fog and main lights of a vehicle, or a light post.
      |
      | For more information, please click Help.
      settings: OpenFcn=open_system([gcb '/Actuator'],'mask')
      mask Help: eval('openHelp(209)')
      mask Display: image(imread('HeadLight.png'))
  TrafficLightRoadSideNL_2_Red : Subsystem  Tag=actuator/Red  Priority=0  LoadFcn=load('PreScanVisuLightActuatorData');load('PrescanRPYData');load('PrescanXYZData');load('PreScanRGBData')  mask(PreScan Sink Block: VisuActiveLight){}
      mask help:
      | The VisuActiveLight block provides a way for detailed animation of Light Sources, such as the indicator, brake, fog and main lights of a vehicle, or a light post.
      |
      | For more information, please click Help.
      settings: OpenFcn=open_system([gcb '/Actuator'],'mask')
      mask Help: eval('openHelp(209)')
      mask Display: image(imread('HeadLight.png'))
  TrafficLightRoadSideNL_3 : Subsystem  Tag=WorldObjectSubSystem  InitFcn=UniqueId = '28';
      mask init: same as PreBraking_Scenario1_cs/TrafficLightRoadSideNL_1
      mask Display: image(imread(imagePath));color('white');text(0, 0, ' ID=14\n')
  TrafficLightRoadSideNL_3_Green : Subsystem  Tag=actuator/Green  Priority=0  LoadFcn=load('PreScanVisuLightActuatorData');load('PrescanRPYData');load('PrescanXYZData');load('PreScanRGBData')  mask(PreScan Sink Block: VisuActiveLight){}
      mask help:
      | The VisuActiveLight block provides a way for detailed animation of Light Sources, such as the indicator, brake, fog and main lights of a vehicle, or a light post.
      |
      | For more information, please click Help.
      settings: OpenFcn=open_system([gcb '/Actuator'],'mask')
      mask Help: eval('openHelp(209)')
      mask Display: image(imread('HeadLight.png'))
  TrafficLightRoadSideNL_3_Orange : Subsystem  Tag=actuator/Orange  Priority=0  LoadFcn=load('PreScanVisuLightActuatorData');load('PrescanRPYData');load('PrescanXYZData');load('PreScanRGBData')  mask(PreScan Sink Block: VisuActiveLight){}
      mask help:
      | The VisuActiveLight block provides a way for detailed animation of Light Sources, such as the indicator, brake, fog and main lights of a vehicle, or a light post.
      |
      | For more information, please click Help.
      settings: OpenFcn=open_system([gcb '/Actuator'],'mask')
      mask Help: eval('openHelp(209)')
      mask Display: image(imread('HeadLight.png'))
  TrafficLightRoadSideNL_3_Red : Subsystem  Tag=actuator/Red  Priority=0  LoadFcn=load('PreScanVisuLightActuatorData');load('PrescanRPYData');load('PrescanXYZData');load('PreScanRGBData')  mask(PreScan Sink Block: VisuActiveLight){}
      mask help:
      | The VisuActiveLight block provides a way for detailed animation of Light Sources, such as the indicator, brake, fog and main lights of a vehicle, or a light post.
      |
      | For more information, please click Help.
      settings: OpenFcn=open_system([gcb '/Actuator'],'mask')
      mask Help: eval('openHelp(209)')
      mask Display: image(imread('HeadLight.png'))
  TrafficLightRoadSideNL_4 : Subsystem  Tag=WorldObjectSubSystem  InitFcn=UniqueId = '29';
      mask init: same as PreBraking_Scenario1_cs/TrafficLightRoadSideNL_1
      mask Display: image(imread(imagePath));color('white');text(0, 0, ' ID=15\n')
  TrafficLightRoadSideNL_4_Green : Subsystem  Tag=actuator/Green  Priority=0  LoadFcn=load('PreScanVisuLightActuatorData');load('PrescanRPYData');load('PrescanXYZData');load('PreScanRGBData')  mask(PreScan Sink Block: VisuActiveLight){}
      mask help:
      | The VisuActiveLight block provides a way for detailed animation of Light Sources, such as the indicator, brake, fog and main lights of a vehicle, or a light post.
      |
      | For more information, please click Help.
      settings: OpenFcn=open_system([gcb '/Actuator'],'mask')
      mask Help: eval('openHelp(209)')
      mask Display: image(imread('HeadLight.png'))
  TrafficLightRoadSideNL_4_Orange : Subsystem  Tag=actuator/Orange  Priority=0  LoadFcn=load('PreScanVisuLightActuatorData');load('PrescanRPYData');load('PrescanXYZData');load('PreScanRGBData')  mask(PreScan Sink Block: VisuActiveLight){}
      mask help:
      | The VisuActiveLight block provides a way for detailed animation of Light Sources, such as the indicator, brake, fog and main lights of a vehicle, or a light post.
      |
      | For more information, please click Help.
      settings: OpenFcn=open_system([gcb '/Actuator'],'mask')
      mask Help: eval('openHelp(209)')
      mask Display: image(imread('HeadLight.png'))
  TrafficLightRoadSideNL_4_Red : Subsystem  Tag=actuator/Red  Priority=0  LoadFcn=load('PreScanVisuLightActuatorData');load('PrescanRPYData');load('PrescanXYZData');load('PreScanRGBData')  mask(PreScan Sink Block: VisuActiveLight){}
      mask help:
      | The VisuActiveLight block provides a way for detailed animation of Light Sources, such as the indicator, brake, fog and main lights of a vehicle, or a light post.
      |
      | For more information, please click Help.
      settings: OpenFcn=open_system([gcb '/Actuator'],'mask')
      mask Help: eval('openHelp(209)')
      mask Display: image(imread('HeadLight.png'))
  WheelL0_Audi_A8_1 : Subsystem  Tag=Actuator  Priority=0  LoadFcn=load('PrescanPoseData');load('PrescanXYZData');load('PreScanRPYData')
      mask help:
      | The VisuJoint block provides a way to adapt the location and orientation of a part of an object.
      |
      | For more information, please click Help.
      settings: OpenFcn=open_system([gcb '/Actuator'],'mask')
      mask Display: image(imread('Joint.png'))
  WheelL0_Citroen_C3_3 : Subsystem  Tag=Actuator  Priority=0  LoadFcn=load('PrescanPoseData');load('PrescanXYZData');load('PreScanRPYData')
      mask help:
      | The VisuJoint block provides a way to adapt the location and orientation of a part of an object.
      |
      | For more information, please click Help.
      settings: OpenFcn=open_system([gcb '/Actuator'],'mask')
      mask Display: image(imread('Joint.png'))
  WheelL0_Toyota_Previa_1 : Subsystem  Tag=Actuator  Priority=0  LoadFcn=load('PrescanPoseData');load('PrescanXYZData');load('PreScanRPYData')
      mask help:
      | The VisuJoint block provides a way to adapt the location and orientation of a part of an object.
      |
      | For more information, please click Help.
      settings: OpenFcn=open_system([gcb '/Actuator'],'mask')
      mask Display: image(imread('Joint.png'))
  WheelL1_Audi_A8_1 : Subsystem  Tag=Actuator  Priority=0  LoadFcn=load('PrescanPoseData');load('PrescanXYZData');load('PreScanRPYData')
      mask help:
      | The VisuJoint block provides a way to adapt the location and orientation of a part of an object.
      |
      | For more information, please click Help.
      settings: OpenFcn=open_system([gcb '/Actuator'],'mask')
      mask Display: image(imread('Joint.png'))
  WheelL1_Citroen_C3_3 : Subsystem  Tag=Actuator  Priority=0  LoadFcn=load('PrescanPoseData');load('PrescanXYZData');load('PreScanRPYData')
      mask help:
      | The VisuJoint block provides a way to adapt the location and orientation of a part of an object.
      |
      | For more information, please click Help.
      settings: OpenFcn=open_system([gcb '/Actuator'],'mask')
      mask Display: image(imread('Joint.png'))
  WheelL1_Toyota_Previa_1 : Subsystem  Tag=Actuator  Priority=0  LoadFcn=load('PrescanPoseData');load('PrescanXYZData');load('PreScanRPYData')
      mask help:
      | The VisuJoint block provides a way to adapt the location and orientation of a part of an object.
      |
      | For more information, please click Help.
      settings: OpenFcn=open_system([gcb '/Actuator'],'mask')
      mask Display: image(imread('Joint.png'))
  WheelR0_Audi_A8_1 : Subsystem  Tag=Actuator  Priority=0  LoadFcn=load('PrescanPoseData');load('PrescanXYZData');load('PreScanRPYData')
      mask help:
      | The VisuJoint block provides a way to adapt the location and orientation of a part of an object.
      |
      | For more information, please click Help.
      settings: OpenFcn=open_system([gcb '/Actuator'],'mask')
      mask Display: image(imread('Joint.png'))
  WheelR0_Citroen_C3_3 : Subsystem  Tag=Actuator  Priority=0  LoadFcn=load('PrescanPoseData');load('PrescanXYZData');load('PreScanRPYData')
      mask help:
      | The VisuJoint block provides a way to adapt the location and orientation of a part of an object.
      |
      | For more information, please click Help.
      settings: OpenFcn=open_system([gcb '/Actuator'],'mask')
      mask Display: image(imread('Joint.png'))
  WheelR0_Toyota_Previa_1 : Subsystem  Tag=Actuator  Priority=0  LoadFcn=load('PrescanPoseData');load('PrescanXYZData');load('PreScanRPYData')
      mask help:
      | The VisuJoint block provides a way to adapt the location and orientation of a part of an object.
      |
      | For more information, please click Help.
      settings: OpenFcn=open_system([gcb '/Actuator'],'mask')
      mask Display: image(imread('Joint.png'))
  WheelR1_Audi_A8_1 : Subsystem  Tag=Actuator  Priority=0  LoadFcn=load('PrescanPoseData');load('PrescanXYZData');load('PreScanRPYData')
      mask help:
      | The VisuJoint block provides a way to adapt the location and orientation of a part of an object.
      |
      | For more information, please click Help.
      settings: OpenFcn=open_system([gcb '/Actuator'],'mask')
      mask Display: image(imread('Joint.png'))
  WheelR1_Citroen_C3_3 : Subsystem  Tag=Actuator  Priority=0  LoadFcn=load('PrescanPoseData');load('PrescanXYZData');load('PreScanRPYData')
      mask help:
      | The VisuJoint block provides a way to adapt the location and orientation of a part of an object.
      |
      | For more information, please click Help.
      settings: OpenFcn=open_system([gcb '/Actuator'],'mask')
      mask Display: image(imread('Joint.png'))
  WheelR1_Toyota_Previa_1 : Subsystem  Tag=Actuator  Priority=0  LoadFcn=load('PrescanPoseData');load('PrescanXYZData');load('PreScanRPYData')
      mask help:
      | The VisuJoint block provides a way to adapt the location and orientation of a part of an object.
      |
      | For more information, please click Help.
      settings: OpenFcn=open_system([gcb '/Actuator'],'mask')
      mask Display: image(imread('Joint.png'))
  wires:
  ToLegacyCollisionOutput/2(Detections) -> Stop Simulation/1  "L2"
  CollisionDetection/1(CollisionDetection) -> ToLegacyCollisionOutput/1(In)
  Citroen_C3_1/1(STATE_Citroen_C3_1_bus) -> STATE_Citroen_C3_1_bus/1(STATE_Citroen_C3_1_bus)
  SELF_Citroen_C3_1/1(SELF_Citroen_C3_1) -> Citroen_C3_1/1(SELF_Citroen_C3_1)
  Ford_Fiesta_1/1(STATE_Ford_Fiesta_1_bus) -> STATE_Ford_Fiesta_1_bus/1(STATE_Ford_Fiesta_1_bus)
  SELF_Ford_Fiesta_1/1(SELF_Ford_Fiesta_1) -> Ford_Fiesta_1/1(SELF_Ford_Fiesta_1)
  Toyota_Yaris_1/1(STATE_Toyota_Yaris_1_bus) -> STATE_Toyota_Yaris_1_bus/1(STATE_Toyota_Yaris_1_bus)
  SELF_Toyota_Yaris_1/1(SELF_Toyota_Yaris_1) -> Toyota_Yaris_1/1(SELF_Toyota_Yaris_1)
  Citroen_C3_2/1(STATE_Citroen_C3_2_bus) -> STATE_Citroen_C3_2_bus/1(STATE_Citroen_C3_2_bus)
  SELF_Citroen_C3_2/1(SELF_Citroen_C3_2) -> Citroen_C3_2/1(SELF_Citroen_C3_2)
  Citroen_C3_3/1(STATE_Citroen_C3_3_bus) -> STATE_Citroen_C3_3_bus/1(STATE_Citroen_C3_3_bus)
  SELF_Citroen_C3_3/1(SELF_Citroen_C3_3) -> Citroen_C3_3/1(SELF_Citroen_C3_3)
  Citroen_C3_3/2(WheelL0_Citroen_C3_3) -> WheelL0_Citroen_C3_3/1(WheelL0_Citroen_C3_3)
  Citroen_C3_3/3(WheelL1_Citroen_C3_3) -> WheelL1_Citroen_C3_3/1(WheelL1_Citroen_C3_3)
  Citroen_C3_3/4(WheelR0_Citroen_C3_3) -> WheelR0_Citroen_C3_3/1(WheelR0_Citroen_C3_3)
  Citroen_C3_3/5(WheelR1_Citroen_C3_3) -> WheelR1_Citroen_C3_3/1(WheelR1_Citroen_C3_3)
  Citroen_C3_3/6(SteeringWheel_Pivot_Citroen_C3_3) -> SteeringWheel_Pivot_Citroen_C3_3/1(SteeringWheel_Pivot_Citroen_C3_3)
  Citroen_C3_3/7(SteeringColumn_Pivot_Citroen_C3_3) -> SteeringColumn_Pivot_Citroen_C3_3/1(SteeringColumn_Pivot_Citroen_C3_3)
  Citroen_C3_3/8(Citroen_C3_3_Brake_light_left) -> Citroen_C3_3_Brake_light_left/1(Citroen_C3_3_Brake_light_left)
  Citroen_C3_3/9(Citroen_C3_3_Brake_light_right) -> Citroen_C3_3_Brake_light_right/1(Citroen_C3_3_Brake_light_right)
  Citroen_C3_3/10(Citroen_C3_3_Indicator_front_left) -> Citroen_C3_3_Indicator_front_left/1(Citroen_C3_3_Indicator_front_left)
  Citroen_C3_3/11(Citroen_C3_3_Indicator_side_left) -> Citroen_C3_3_Indicator_side_left/1(Citroen_C3_3_Indicator_side_left)
  Citroen_C3_3/12(Citroen_C3_3_Indicator_rear_left) -> Citroen_C3_3_Indicator_rear_left/1(Citroen_C3_3_Indicator_rear_left)
  Citroen_C3_3/13(Citroen_C3_3_Indicator_front_right) -> Citroen_C3_3_Indicator_front_right/1(Citroen_C3_3_Indicator_front_right)
  Citroen_C3_3/14(Citroen_C3_3_Indicator_side_right) -> Citroen_C3_3_Indicator_side_right/1(Citroen_C3_3_Indicator_side_right)
  Citroen_C3_3/15(Citroen_C3_3_Indicator_rear_right) -> Citroen_C3_3_Indicator_rear_right/1(Citroen_C3_3_Indicator_rear_right)
  Toyota_Previa_1/1(STATE_Toyota_Previa_1_bus) -> STATE_Toyota_Previa_1_bus/1(STATE_Toyota_Previa_1_bus)
  SELF_Toyota_Previa_1/1(SELF_Toyota_Previa_1) -> Toyota_Previa_1/1(SELF_Toyota_Previa_1)
  Toyota_Previa_1/2(WheelL0_Toyota_Previa_1) -> WheelL0_Toyota_Previa_1/1(WheelL0_Toyota_Previa_1)
  Toyota_Previa_1/3(WheelL1_Toyota_Previa_1) -> WheelL1_Toyota_Previa_1/1(WheelL1_Toyota_Previa_1)
  Toyota_Previa_1/4(WheelR0_Toyota_Previa_1) -> WheelR0_Toyota_Previa_1/1(WheelR0_Toyota_Previa_1)
  Toyota_Previa_1/5(WheelR1_Toyota_Previa_1) -> WheelR1_Toyota_Previa_1/1(WheelR1_Toyota_Previa_1)
  Toyota_Previa_1/6(SteeringWheel_pivot_Toyota_Previa_1) -> SteeringWheel_pivot_Toyota_Previa_1/1(SteeringWheel_pivot_Toyota_Previa_1)
  Toyota_Previa_1/7(SteeringColumn_pivot_Toyota_Previa_1) -> SteeringColumn_pivot_Toyota_Previa_1/1(SteeringColumn_pivot_Toyota_Previa_1)
  Toyota_Previa_1/8(Toyota_Previa_1_Brake_light_center) -> Toyota_Previa_1_Brake_light_center/1(Toyota_Previa_1_Brake_light_center)
  Toyota_Previa_1/9(Toyota_Previa_1_Brake_light_left) -> Toyota_Previa_1_Brake_light_left/1(Toyota_Previa_1_Brake_light_left)
  Toyota_Previa_1/10(Toyota_Previa_1_Brake_light_right) -> Toyota_Previa_1_Brake_light_right/1(Toyota_Previa_1_Brake_light_right)
  Toyota_Previa_1/11(Toyota_Previa_1_Indicator_front_left) -> Toyota_Previa_1_Indicator_front_left/1(Toyota_Previa_1_Indicator_front_left)
  Toyota_Previa_1/12(Toyota_Previa_1_Indicator_side_left) -> Toyota_Previa_1_Indicator_side_left/1(Toyota_Previa_1_Indicator_side_left)
  Toyota_Previa_1/13(Toyota_Previa_1_Indicator_rear_left) -> Toyota_Previa_1_Indicator_rear_left/1(Toyota_Previa_1_Indicator_rear_left)
  Toyota_Previa_1/14(Toyota_Previa_1_Indicator_front_right) -> Toyota_Previa_1_Indicator_front_right/1(Toyota_Previa_1_Indicator_front_right)
  Toyota_Previa_1/15(Toyota_Previa_1_Indicator_side_right) -> Toyota_Previa_1_Indicator_side_right/1(Toyota_Previa_1_Indicator_side_right)
  Toyota_Previa_1/16(Toyota_Previa_1_Indicator_rear_right) -> Toyota_Previa_1_Indicator_rear_right/1(Toyota_Previa_1_Indicator_rear_right)
  Audi_A8_1/1(STATE_Audi_A8_1_bus) -> STATE_Audi_A8_1_bus/1(STATE_Audi_A8_1_bus)
  SELF_Audi_A8_1/1(SELF_Audi_A8_1) -> Audi_A8_1/1(SELF_Audi_A8_1)
  TIS_1/1(TIS_1) -> Audi_A8_1/2(TIS_1)
  TIS_2/1(TIS_2) -> Audi_A8_1/3(TIS_2)
  Audi_A8_1/2(WheelL0_Audi_A8_1) -> WheelL0_Audi_A8_1/1(WheelL0_Audi_A8_1)
  Audi_A8_1/3(WheelL1_Audi_A8_1) -> WheelL1_Audi_A8_1/1(WheelL1_Audi_A8_1)
  Audi_A8_1/4(WheelR0_Audi_A8_1) -> WheelR0_Audi_A8_1/1(WheelR0_Audi_A8_1)
  Audi_A8_1/5(WheelR1_Audi_A8_1) -> WheelR1_Audi_A8_1/1(WheelR1_Audi_A8_1)
  Audi_A8_1/6(SteeringWheel_pivot_Audi_A8_1) -> SteeringWheel_pivot_Audi_A8_1/1(SteeringWheel_pivot_Audi_A8_1)
  Audi_A8_1/7(SteeringColumn_pivot_Audi_A8_1) -> SteeringColumn_pivot_Audi_A8_1/1(SteeringColumn_pivot_Audi_A8_1)
  Audi_A8_1/8(Audi_A8_1_Brake_light_left) -> Audi_A8_1_Brake_light_left/1(Audi_A8_1_Brake_light_left)
  Audi_A8_1/9(Audi_A8_1_Brake_light_right) -> Audi_A8_1_Brake_light_right/1(Audi_A8_1_Brake_light_right)
  Audi_A8_1/10(Audi_A8_1_Indicator_front_left) -> Audi_A8_1_Indicator_front_left/1(Audi_A8_1_Indicator_front_left)
  Audi_A8_1/11(Audi_A8_1_Indicator_rear_left) -> Audi_A8_1_Indicator_rear_left/1(Audi_A8_1_Indicator_rear_left)
  Audi_A8_1/12(Audi_A8_1_Indicator_front_right) -> Audi_A8_1_Indicator_front_right/1(Audi_A8_1_Indicator_front_right)
  Audi_A8_1/13(Audi_A8_1_Indicator_rear_right) -> Audi_A8_1_Indicator_rear_right/1(Audi_A8_1_Indicator_rear_right)
  Sphere_1/1(STATE_Sphere_1_bus) -> STATE_Sphere_1_bus/1(STATE_Sphere_1_bus)
  SELF_Sphere_1/1(SELF_Sphere_1) -> Sphere_1/1(SELF_Sphere_1)
  TrafficLightRoadSideNL_1/1(TrafficLightRoadSideNL_1_Red) -> TrafficLightRoadSideNL_1_Red/1(TrafficLightRoadSideNL_1_Red)
  TrafficLightRoadSideNL_1/2(TrafficLightRoadSideNL_1_Orange) -> TrafficLightRoadSideNL_1_Orange/1(TrafficLightRoadSideNL_1_Orange)
  TrafficLightRoadSideNL_1/3(TrafficLightRoadSideNL_1_Green) -> TrafficLightRoadSideNL_1_Green/1(TrafficLightRoadSideNL_1_Green)
  TrafficLightRoadSideNL_2/1(TrafficLightRoadSideNL_2_Red) -> TrafficLightRoadSideNL_2_Red/1(TrafficLightRoadSideNL_2_Red)
  TrafficLightRoadSideNL_2/2(TrafficLightRoadSideNL_2_Orange) -> TrafficLightRoadSideNL_2_Orange/1(TrafficLightRoadSideNL_2_Orange)
  TrafficLightRoadSideNL_2/3(TrafficLightRoadSideNL_2_Green) -> TrafficLightRoadSideNL_2_Green/1(TrafficLightRoadSideNL_2_Green)
  TrafficLightRoadSideNL_3/1(TrafficLightRoadSideNL_3_Red) -> TrafficLightRoadSideNL_3_Red/1(TrafficLightRoadSideNL_3_Red)
  TrafficLightRoadSideNL_3/2(TrafficLightRoadSideNL_3_Orange) -> TrafficLightRoadSideNL_3_Orange/1(TrafficLightRoadSideNL_3_Orange)
  TrafficLightRoadSideNL_3/3(TrafficLightRoadSideNL_3_Green) -> TrafficLightRoadSideNL_3_Green/1(TrafficLightRoadSideNL_3_Green)
  TrafficLightRoadSideNL_4/1(TrafficLightRoadSideNL_4_Red) -> TrafficLightRoadSideNL_4_Red/1(TrafficLightRoadSideNL_4_Red)
  TrafficLightRoadSideNL_4/2(TrafficLightRoadSideNL_4_Orange) -> TrafficLightRoadSideNL_4_Orange/1(TrafficLightRoadSideNL_4_Orange)
  TrafficLightRoadSideNL_4/3(TrafficLightRoadSideNL_4_Green) -> TrafficLightRoadSideNL_4_Green/1(TrafficLightRoadSideNL_4_Green)
  ToLegacyCollisionOutput/1(IDs) -> Terminator_1/1
